simulink model "VGWEC_Model_Final"  (R2022a)
settings: Solver=ode3  StartTime=0.0  StopTime=tSim  FixedStep=dt  RelTol=1e-3
undefined symbols (not defined in the file): amp_Wave, AR3, aRInterp, BR3, bRInterp, CR3, DR3, hydroCoeff, hydroVCoeff, I55, tfRadAR_ROm, tfRadBR_ROm, tfRadCR_ROm, tfRadDR_ROm, theta0, Time_Variant, tRamp, w_Wave, w_WaveIndx, X, Y, Z
libraries: sm_lib x8, nesl_utility x5, cstblocks x4, simulink x2
settings Model: Creator=tdemonte  LastModifiedBy=tdemonte
settings SimscapeCC: EditingMode=Restricted
settings ExplorerConfigSet: InternalSimMechanicsExplorerSettings="<ExplorerConfiguration><canonicalview>default</canonicalview><AnimationSetting><BasePlaybackSpeed>1.0</BasePlaybackSpeed><PlaybackSpeedFactor>1.0</PlaybackSpeedFactor></AnimationSetting><TilePanel><TileInfo><Tiles Columns=\"1\" Count=\"1\" Rows=\"1\"><Column Weight=\"1\"/><Row Weight=\"1\"/><Tile Height=\"1\" Width=\"1\" X=\"0\" Y=\"0\"/></Tiles></TileInfo><SceneInfo><SceneViewer><BGColor><R>0.800000011920928955</R><G>0.800000011920928955</G><B>0.800000011920928955</B></BGColor><Camera><DoPerspective>off</DoPerspective><Position><X>1.56106141432910372</X><Y>-1.5610514773575217</Y><Z>1.56105459035981609</Z></Position><Center><X>9.99552486290526904e-06</X><Y>-5.85532809332417288e-08</Y><Z>3.17155557533474546e-06</Z></Center><Up><X>-0.408248290463863073</X><Y>0.408248290463863073</Y><Z>0.816496580927726145</Z></Up><ViewLimDist>1</ViewLimDist><YLim>1.9911708307266236</YLim><XLim>3.77091781730319342</XLim></Camera></SceneViewer></SceneInfo></TilePanel><MechEditorPanel><Cameras/><GfxPanelCameraMap/><VideoCreator><PlaybackSpeedRatio>1.0</PlaybackSpeedRatio><FrameRate>30</FrameRate><VideoFormat>Motion JPEG AVI</VideoFormat><FrameSize>auto</FrameSize></VideoCreator></MechEditorPanel></ExplorerConfiguration>"

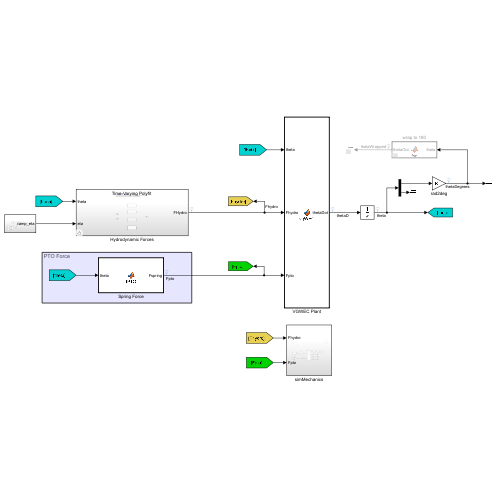
[thumbnail: Simulink's stored preview of the top-level diagram]
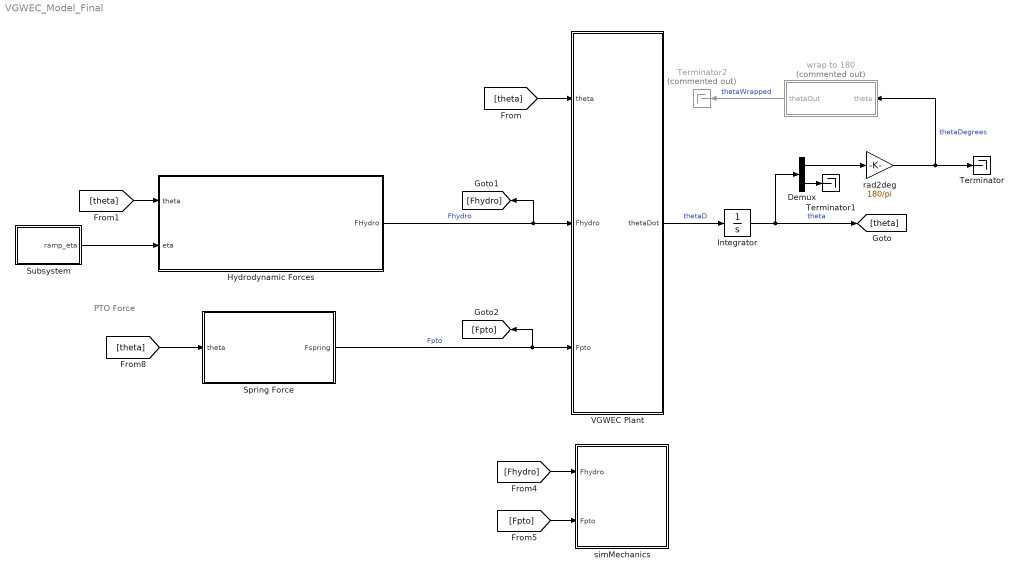
== system VGWEC_Model_Final ==
  note: PTO Force
  Demux : Demux  Outputs=2
  Hydrodynamic Forces : Subsystem  Variant=on
  Integrator : Integrator  InitialCondition=theta0
  Spring Force : MATLAB Function  TreatAsAtomicUnit=on
  Subsystem : Subsystem
  Terminator : Terminator
  Terminator1 : Terminator
  Terminator2 : Terminator  Commented=on
  VGWEC Plant : MATLAB Function  TreatAsAtomicUnit=on
  rad2deg : Gain  Gain=180/pi
  simMechanics : Subsystem
  wrap to 180 : MATLAB Function  Commented=on  TreatAsAtomicUnit=on
  wires:
  VGWEC Plant/1(thetaDot) -> Integrator/1  "thetaD"
  [theta] -> VGWEC Plant/1(theta)
  rad2deg/1 -> Terminator/1, wrap to 180/1(theta)  "thetaDegrees"
  [theta] -> Spring Force/1(theta)
  Spring Force/1(Fspring) -> [Fpto], VGWEC Plant/3(Fpto)  "Fpto"
  [theta] -> Hydrodynamic Forces/1(theta)
  Hydrodynamic Forces/1(FHydro) -> [Fhydro], VGWEC Plant/2(Fhydro)  "Fhydro"
  [Fhydro] -> simMechanics/1(Fhydro)
  [Fpto] -> simMechanics/2(Fpto)
  Integrator/1 -> Demux/1, [theta]  "theta"
  Subsystem/1(ramp_eta) -> Hydrodynamic Forces/2(eta)
  Demux/1 -> rad2deg/1
  Demux/2 -> Terminator1/1
  wrap to 180/1(thetaOut) -> Terminator2/1  "thetaWrapped"

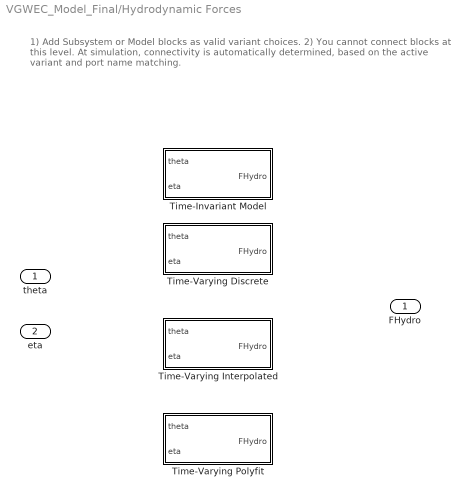
== system VGWEC_Model_Final/Hydrodynamic Forces ==
  note: 1) Add Subsystem or Model blocks as valid variant choices.
      | 2) You cannot connect blocks at this level. At simulation, connectivity is automatically
      | determined, based on the active variant and port name matching.
  theta : Inport
  eta : Inport  Port=2
  Time-Invariant Model : Subsystem  VariantControl=Time_Variant == 0
  "Time-Varying Discrete " : Subsystem  VariantControl=Time_Variant == 1
  Time-Varying Interpolated : Subsystem  VariantControl=Time_Variant == 2
  "Time-Varying Polyfit " : Subsystem  VariantControl=Time_Variant == 3
  FHydro : Outport

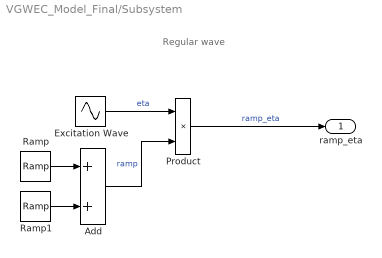
== system VGWEC_Model_Final/Subsystem ==
  note: Regular wave
  Add : Sum
  Excitation Wave : Sin  Amplitude=amp_Wave  Frequency=w_Wave  SampleTime=0
  Product : Product
  Ramp : simulink/Sources/Ramp  slope=1/tRamp  start=0  InitialOutput=0
  Ramp1 : simulink/Sources/Ramp  slope=-1/tRamp  start=tRamp  InitialOutput=0
  ramp_eta : Outport
  wires:
  Add/1 -> Product/2  "ramp"
  Excitation Wave/1 -> Product/1  "eta"
  Ramp1/1 -> Add/2
  Product/1 -> ramp_eta/1  "ramp_eta"
  Ramp/1 -> Add/1

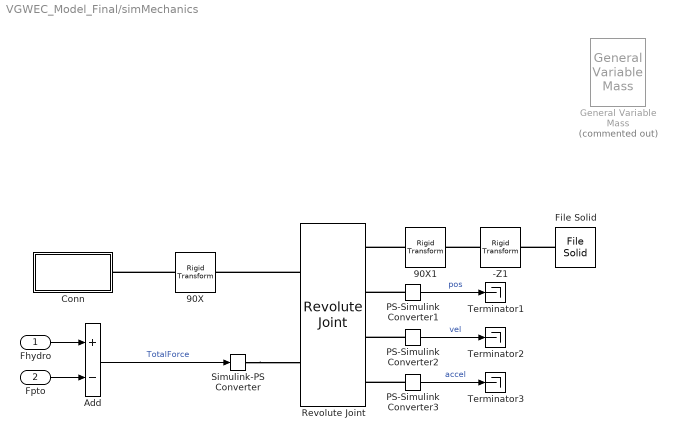
== system VGWEC_Model_Final/simMechanics ==
  Fhydro : Inport
  Fpto : Inport  Port=2
  -Z1 : sm_lib/Frames and Transforms/Rigid Transform  TranslationMethod=StandardAxis  TranslationStandardOffset=1  TranslationLengthUnit=m  TranslationStandardAxis=+Z  TranslationCartesianOffset=[0 0 ]  TranslationROffset=0  TranslationROffsetUnits=m  TranslationZOffset=0  TranslationZOffsetUnits=m  TranslationThetaOffset=0  TranslationThetaOffsetUnits=deg  RotationMethod=None  RotationAngleUnits=deg  RotationStandardAxis=+X  RotationAngle=90  RotationArbitraryAxis=[0 0 1]  FollAlignAxisA=+X  BaseAlignAxisA=+Y  FollAlignAxisB=+Y  BaseAlignAxisB=+Z  RotationSequenceAxes=FollowerAxes  RotationSequence=XYX  RotationSequenceAngles=[0 0 0]  RotationSequenceAnglesUnits=deg  RotationMatrix=[1 0 0; 0 1 0; 0 0 1]
  90X : sm_lib/Frames and Transforms/Rigid Transform  TranslationMethod=None  TranslationStandardOffset=1  TranslationLengthUnit=m  TranslationStandardAxis=-Y  TranslationCartesianOffset=[0 0 ]  TranslationROffset=0  TranslationROffsetUnits=m  TranslationZOffset=0  TranslationZOffsetUnits=m  TranslationThetaOffset=0  TranslationThetaOffsetUnits=deg  RotationMethod=StandardAxis  RotationAngleUnits=deg  RotationStandardAxis=+X  RotationAngle=90  RotationArbitraryAxis=[0 0 1]  FollAlignAxisA=+X  BaseAlignAxisA=+Y  FollAlignAxisB=+Y  BaseAlignAxisB=+Z  RotationSequenceAxes=FollowerAxes  RotationSequence=XYX  RotationSequenceAngles=[0 0 0]  RotationSequenceAnglesUnits=deg  RotationMatrix=[1 0 0; 0 1 0; 0 0 1]
  90X1 : sm_lib/Frames and Transforms/Rigid Transform  TranslationMethod=None  TranslationStandardOffset=0  TranslationLengthUnit=m  TranslationStandardAxis=+Z  TranslationCartesianOffset=[0 -1 0]  TranslationROffset=0  TranslationROffsetUnits=m  TranslationZOffset=0  TranslationZOffsetUnits=m  TranslationThetaOffset=0  TranslationThetaOffsetUnits=deg  RotationMethod=StandardAxis  RotationAngleUnits=deg  RotationStandardAxis=-X  RotationAngle=90  RotationArbitraryAxis=[0 0 1]  FollAlignAxisA=+X  BaseAlignAxisA=+Y  FollAlignAxisB=+Y  BaseAlignAxisB=+Z  RotationSequenceAxes=FollowerAxes  RotationSequence=XYX  RotationSequenceAngles=[0 0 0]  RotationSequenceAnglesUnits=deg  RotationMatrix=[1 0 0; 0 1 0; 0 0 1]
  Add : Sum  Inputs=+-
  Conn : Subsystem
  File Solid : sm_lib/Body Elements/File Solid  ExtGeomFileName=C:\Users\tdemonte\OneDrive - NREL\VGWEC\Full Flap Data\flap0deg.STL  UnitType=Custom  ExtGeomFileUnits=mm  StepReaderType=HEX  ExportConvexHullGeometry=off  InertiaType=Custom  Mass=I55  MassUnits=kg  CenterOfMass=[0 0 -1]  CenterOfMassUnits=m  MomentsOfInertia=[1 hydroVCoeff.IA(hydroCoeff.singleThetaIndex) + hydroCoeff.IQ 1]  MomentsOfInertiaUnits=kg*m^2  ProductsOfInertia=[0 0 0]  ProductsOfInertiaUnits=kg*m^2  BasedOnType=Mass  Density=1000  DensityUnits=kg/m^3  DoExposeReferenceFrame=on  SerializedFrames=<Frames/>  GraphicType=FromGeometry  MarkerShape=Sphere  MarkerSize=10  GraphicVisPropType=SimpleVisualProperties  GraphicDiffuseColor=[0.5 0.5 0.5]  GraphicSpecularColor=[0.5 0.5 0.5 1.0]  GraphicAmbientColor=[0.15 0.15 0.15 1.0]  GraphicEmissiveColor=[0.0 0.0 0.0 1.0]  GraphicShininess=75  GraphicOpacity=0.5
  General Variable Mass : sm_lib/Body Elements/Variable Mass/General Variable Mass  Commented=on  VariableInertiaType=Custom  MassType=TimeVarying  Mass=1  MassUnits=kg  CenterOfMassType=Constant  CenterOfMass=[0 0 0]  CenterOfMassUnits=m  InertiaMatrixType=Constant  MomentsOfInertia=[1 1 1]  MomentsOfInertiaUnits=kg*m^2  ProductsOfInertia=[0 0 0]  ProductsOfInertiaUnits=kg*m^2  GraphicType=InertiaEllipsoid  MarkerShape=Sphere  MarkerSize=10  GraphicVisPropType=SimpleVisualProperties  GraphicDiffuseColor=[0.5 0.5 0.5]  GraphicSpecularColor=[0.5 0.5 0.5 1.0]  GraphicAmbientColor=[0.15 0.15 0.15 1.0]  GraphicEmissiveColor=[0.0 0.0 0.0 1.0]  GraphicShininess=75  GraphicOpacity=1.0
      settings: SourceProductBaseCode=MS
  PS-Simulink Converter1 : nesl_utility/PS-Simulink Converter  PhysicalDomain=network_engine_domain  SubClassName=ps_output  LeftPortType=input  RightPortType=output  PseudoPeriodic=off  Frequencies=[]  VectorFormat=inherit  Unit=inherit  AffineConversion=off
      settings: SourceProductBaseCode=SS,PW,VE
  PS-Simulink Converter2 : nesl_utility/PS-Simulink Converter  PhysicalDomain=network_engine_domain  SubClassName=ps_output  LeftPortType=input  RightPortType=output  PseudoPeriodic=off  Frequencies=[]  VectorFormat=inherit  Unit=inherit  AffineConversion=off
      settings: SourceProductBaseCode=SS,PW,VE
  PS-Simulink Converter3 : nesl_utility/PS-Simulink Converter  PhysicalDomain=network_engine_domain  SubClassName=ps_output  LeftPortType=input  RightPortType=output  PseudoPeriodic=off  Frequencies=[]  VectorFormat=inherit  Unit=inherit  AffineConversion=off
      settings: SourceProductBaseCode=SS,PW,VE
  Revolute Joint : sm_lib/Joints/Revolute Joint  JointMode=Normal  SenseConstraintForce=off  SenseConstraintForceX=off  SenseConstraintForceY=off  SenseConstraintForceZ=off  SenseConstraintTorque=off  SenseConstraintTorqueX=off  SenseConstraintTorqueY=off  SenseConstraintTorqueZ=off  SenseTotalForce=off  SenseTotalForceX=off  SenseTotalForceY=off  SenseTotalForceZ=off  SenseTotalTorque=off  SenseTotalTorqueX=off  SenseTotalTorqueY=off  SenseTotalTorqueZ=off  CompositeWrenchDir=FollowerOnBase  CompositeWrenchFrame=BaseFrame  EquilibriumPosition=0  EquilibriumPositionUnits=deg  SpringStiffness=0  SpringStiffnessUnits=N*m/deg  DampingCoefficient=0  DampingCoefficientUnits=N*m/(deg/s)  TorqueActuationMode=InputTorque  MotionActuationMode=ComputedMotion  SensePosition=on  SenseVelocity=on  SenseAcceleration=on  SenseTorqueForce=off  SenseLowerLimitTorqueForce=off  SenseUpperLimitTorqueForce=off  LowerLimitSpecify=off  LowerLimitBound=-90  LowerLimitBoundUnits=deg  LowerLimitStiffness=1e4  LowerLimitStiffnessUnits=N*m/deg  LowerLimitDamping=10  LowerLimitDampingUnits=N*m/(deg/s)  LowerLimitTransitionRegionWidth=0.1  LowerLimitTransitionRegionWidthUnits=deg  UpperLimitSpecify=off  UpperLimitBound=90  UpperLimitBoundUnits=deg  UpperLimitStiffness=1e4  UpperLimitStiffnessUnits=N*m/deg  UpperLimitDamping=10  UpperLimitDampingUnits=N*m/(deg/s)  UpperLimitTransitionRegionWidth=0.1  UpperLimitTransitionRegionWidthUnits=deg  PositionTargetSpecify=off  PositionTargetPriority=High  PositionTargetValue=0  PositionTargetValueUnits=deg  VelocityTargetSpecify=off  VelocityTargetPriority=High  VelocityTargetValue=0  VelocityTargetValueUnits=deg/s
  Simulink-PS Converter : nesl_utility/Simulink-PS Converter  PhysicalDomain=network_engine_domain  SubClassName=ps_input  LeftPortType=input  RightPortType=output  PseudoPeriodic=off  Frequencies=[]  NoiseDistribution=none  NoiseParameters=[]  Unit=1  AffineConversion=off  FilteringAndDerivatives=provide  SimscapeFilterOrder=1  InputFilterTimeConstant=0.001  UdotUserProvided=0
      settings: SourceProductBaseCode=SS,PW,VE
  Terminator1 : Terminator
  Terminator2 : Terminator
  Terminator3 : Terminator
  wires:
  Add/1 -> Simulink-PS Converter/1  "TotalForce"
  PS-Simulink Converter3/1 -> Terminator3/1  "accel"
  PS-Simulink Converter2/1 -> Terminator2/1  "vel"
  PS-Simulink Converter1/1 -> Terminator1/1  "pos"
  Fhydro/1 -> Add/1
  Fpto/1 -> Add/2
  connections:
  PS-Simulink Converter3/LConn1 -- Revolute Joint/RConn4
  File Solid/RConn1 -- -Z1/RConn1
  PS-Simulink Converter2/LConn1 -- Revolute Joint/RConn3
  PS-Simulink Converter1/LConn1 -- Revolute Joint/RConn2
  Simulink-PS Converter/RConn1 -- Revolute Joint/LConn2
  Revolute Joint/LConn1 -- 90X/RConn1
  90X1/LConn1 -- Revolute Joint/RConn1
  90X/LConn1 -- Conn/RConn1
  -Z1/LConn1 -- 90X1/RConn1

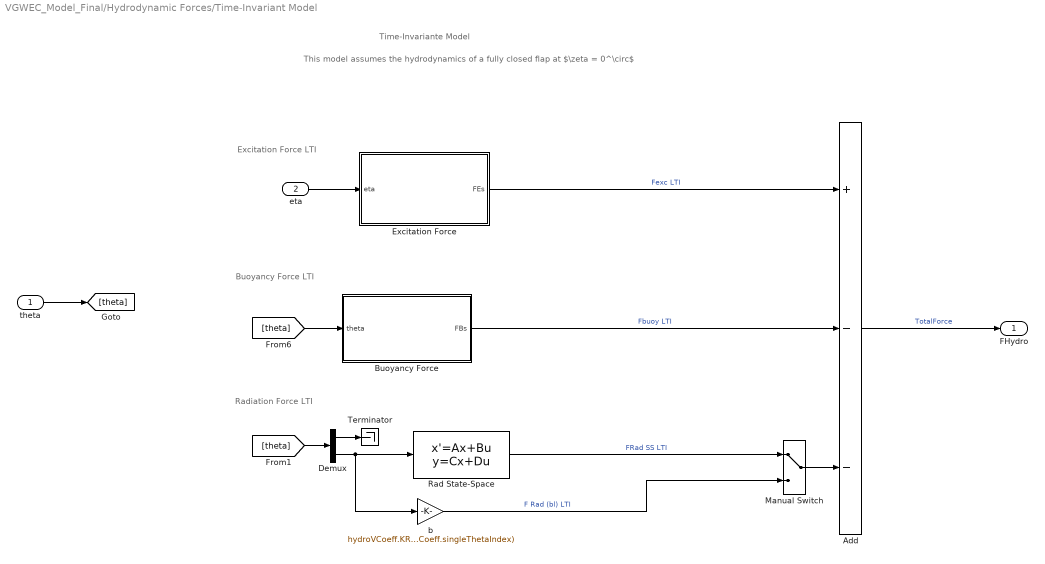
== system VGWEC_Model_Final/Hydrodynamic Forces/Time-Invariant Model ==
  note: Time-Invariante Model
  note: Excitation Force LTI
  note: Radiation Force LTI
  note: Buoyancy Force LTI
  note: This model assumes the hydrodynamics of a fully closed flap at $\zeta = 0^\circ$
  theta : Inport
  eta : Inport  Port=2
  Add : Sum  Inputs=+--
  Buoyancy Force : MATLAB Function  TreatAsAtomicUnit=on
  Demux : Demux  Outputs=2
  "Excitation Force " : MATLAB Function  TreatAsAtomicUnit=on
  Manual Switch : ManualSwitch
  Rad State-Space : StateSpace  A=AR3  B=BR3  C=CR3  D=DR3  InitialCondition=0
  Terminator : Terminator
  b : Gain  Gain=hydroVCoeff.KR(w_WaveIndx, hydroCoeff.singleThetaIndex)
  FHydro : Outport
  wires:
  "Excitation Force "/1(FEs) -> Add/1  "Fexc LTI"
  Demux/2 -> b/1, Rad State-Space/1
  Buoyancy Force/1(FBs) -> Add/2  "Fbuoy LTI"
  eta/1 -> "Excitation Force "/1(eta)
  theta/1 -> [theta]
  [theta] -> Buoyancy Force/1(theta)
  Rad State-Space/1 -> Manual Switch/1  "FRad SS LTI"
  Demux/1 -> Terminator/1
  [theta] -> Demux/1
  Add/1 -> FHydro/1  "TotalForce"
  b/1 -> Manual Switch/2  "F Rad (bl) LTI"
  Manual Switch/1 -> Add/3

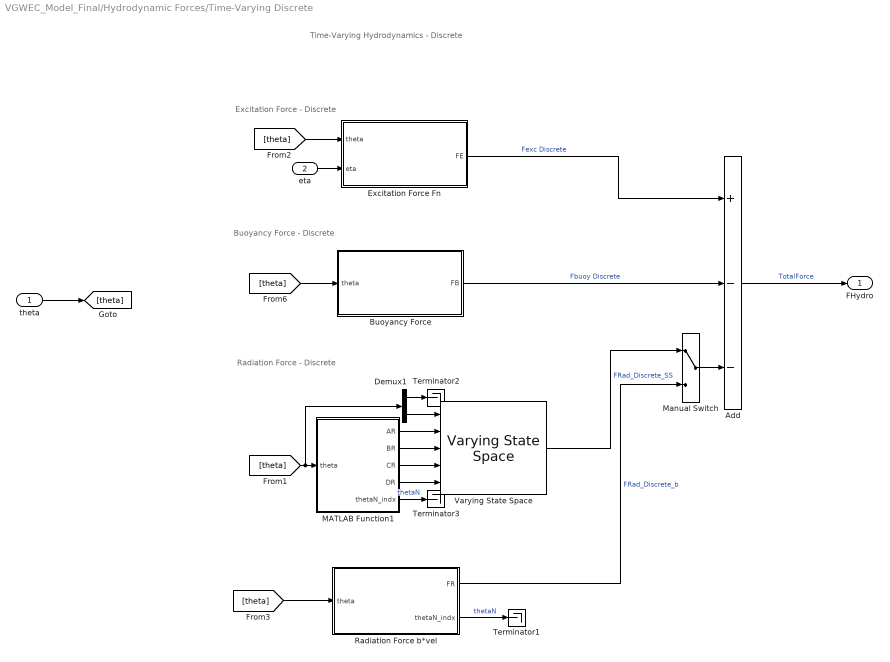
== system VGWEC_Model_Final/Hydrodynamic Forces/Time-Varying Discrete  ==
  note: Buoyancy Force - Discrete
  note: Excitation Force - Discrete
  note: Time-Varying Hydrodynamics - Discrete
  note: Radiation Force - Discrete
  theta : Inport
  eta : Inport  Port=2
  Add : Sum  Inputs=+--
  Buoyancy Force : MATLAB Function  TreatAsAtomicUnit=on
  Demux1 : Demux  Outputs=2
  Excitation Force Fn : MATLAB Function  TreatAsAtomicUnit=on
  MATLAB Function1 : MATLAB Function  TreatAsAtomicUnit=on
  Manual Switch : ManualSwitch
  Radiation Force b*vel : MATLAB Function  TreatAsAtomicUnit=on
  Terminator1 : Terminator
  Terminator2 : Terminator
  Terminator3 : Terminator
  Varying State Space : cstblocks/Linear Parameter Varying/Varying State Space  x0=0  xNames=''  OutputX=off  OutputDX=off
  FHydro : Outport
  wires:
  eta/1 -> Excitation Force Fn/2(eta)
  Buoyancy Force/1(FB) -> Add/2  "Fbuoy Discrete"
  Excitation Force Fn/1(FE) -> Add/1  "Fexc Discrete"
  Add/1 -> FHydro/1  "TotalForce"
  theta/1 -> [theta]
  [theta] -> Excitation Force Fn/1(theta)
  [theta] -> Buoyancy Force/1(theta)
  Demux1/2 -> Varying State Space/1
  Varying State Space/1 -> Manual Switch/1  "FRad_Discrete_SS"
  [theta] -> Demux1/1, MATLAB Function1/1(theta)
  [theta] -> Radiation Force b*vel/1(theta)
  MATLAB Function1/5(thetaN_indx) -> Terminator3/1  "thetaN"
  MATLAB Function1/2(BR) -> Varying State Space/3
  MATLAB Function1/1(AR) -> Varying State Space/2
  MATLAB Function1/3(CR) -> Varying State Space/4
  Radiation Force b*vel/1(FR) -> Manual Switch/2  "FRad_Discrete_b"
  Demux1/1 -> Terminator2/1
  MATLAB Function1/4(DR) -> Varying State Space/5
  Manual Switch/1 -> Add/3
  Radiation Force b*vel/2(thetaN_indx) -> Terminator1/1  "thetaN"

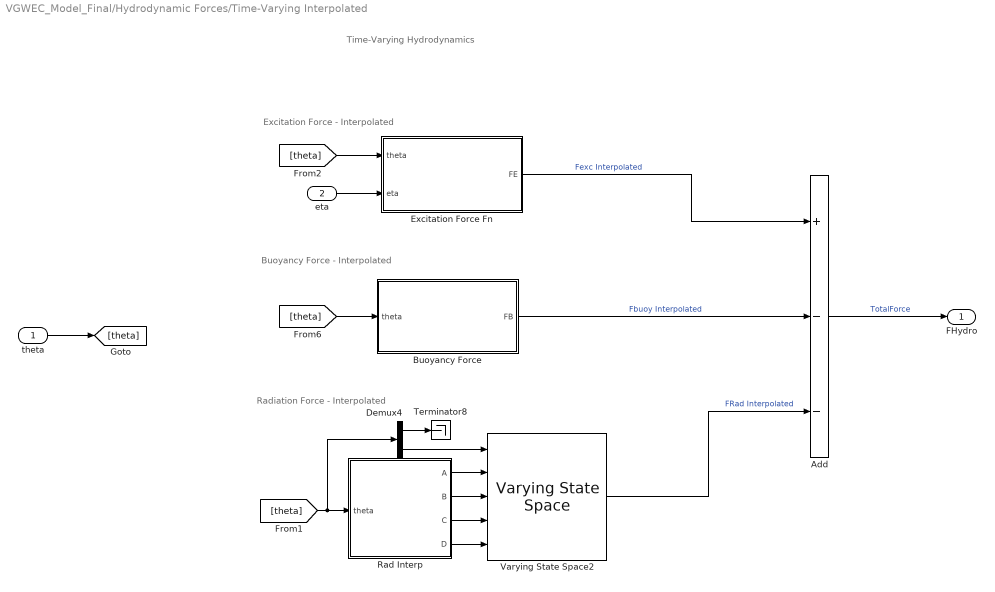
== system VGWEC_Model_Final/Hydrodynamic Forces/Time-Varying Interpolated ==
  note: Radiation Force - Interpolated
  note: Time-Varying Hydrodynamics
  note: Excitation Force - Interpolated
  note: Buoyancy Force - Interpolated
  theta : Inport
  eta : Inport  Port=2
  Add : Sum  Inputs=+--
  Buoyancy Force : MATLAB Function  TreatAsAtomicUnit=on
  Demux4 : Demux  Outputs=2
  Excitation Force Fn : MATLAB Function  TreatAsAtomicUnit=on
  Rad Interp : MATLAB Function  TreatAsAtomicUnit=on
  Terminator8 : Terminator
  Varying State Space2 : cstblocks/Linear Parameter Varying/Varying State Space  x0=0  xNames=''  OutputX=off  OutputDX=off
  FHydro : Outport
  wires:
  [theta] -> Buoyancy Force/1(theta)
  [theta] -> Excitation Force Fn/1(theta)
  theta/1 -> [theta]
  Add/1 -> FHydro/1  "TotalForce"
  Excitation Force Fn/1(FE) -> Add/1  "Fexc Interpolated"
  Buoyancy Force/1(FB) -> Add/2  "Fbuoy Interpolated"
  eta/1 -> Excitation Force Fn/2(eta)
  Demux4/2 -> Varying State Space2/1
  Rad Interp/3(C) -> Varying State Space2/4
  Rad Interp/1(A) -> Varying State Space2/2
  Demux4/1 -> Terminator8/1
  Rad Interp/2(B) -> Varying State Space2/3
  Rad Interp/4(D) -> Varying State Space2/5
  [theta] -> Demux4/1, Rad Interp/1(theta)
  Varying State Space2/1 -> Add/3  "FRad Interpolated"

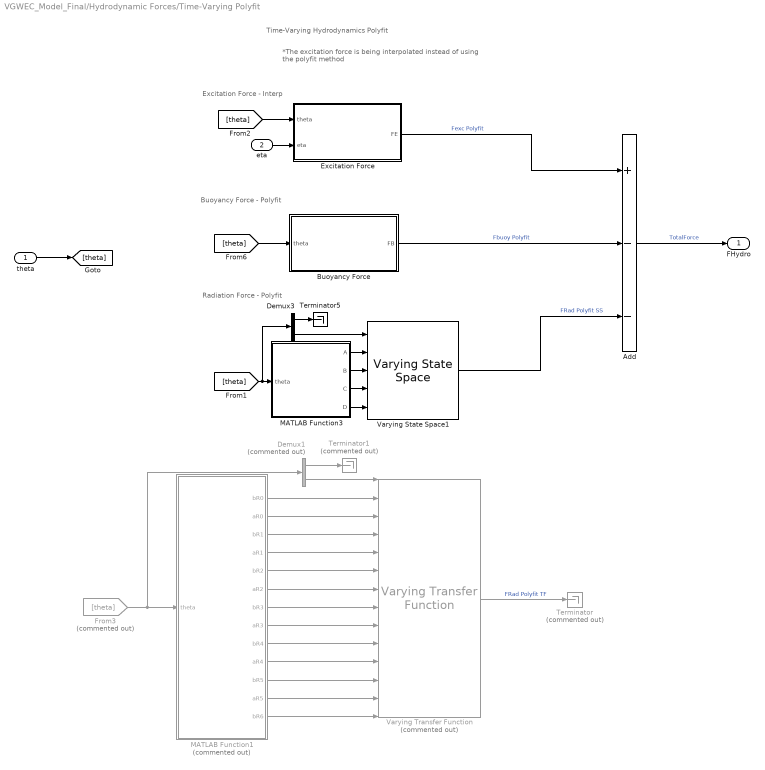
== system VGWEC_Model_Final/Hydrodynamic Forces/Time-Varying Polyfit  ==
  note: Radiation Force - Polyfit
  note: Time-Varying Hydrodynamics Polyfit
  note: Excitation Force - Interp
  note: Buoyancy Force - Polyfit
  note: *The excitation force is being interpolated instead of using the polyfit method
  theta : Inport
  eta : Inport  Port=2
  Add : Sum  Inputs=+--
  Buoyancy Force : MATLAB Function  TreatAsAtomicUnit=on
  Demux1 : Demux  Commented=on  Outputs=2
  Demux3 : Demux  Outputs=2
  Excitation Force : MATLAB Function  TreatAsAtomicUnit=on
  From3 : From  Commented=on  GotoTag=theta
  MATLAB Function1 : MATLAB Function  Commented=on  TreatAsAtomicUnit=on
  MATLAB Function3 : MATLAB Function  TreatAsAtomicUnit=on
  Terminator : Terminator  Commented=on
  Terminator1 : Terminator  Commented=on
  Terminator5 : Terminator
  Varying State Space1 : cstblocks/Linear Parameter Varying/Varying State Space  x0=0  xNames=''  OutputX=off  OutputDX=off
  Varying Transfer Function : cstblocks/Linear Parameter Varying/Varying Transfer Function  Commented=on  N=6
  FHydro : Outport
  wires:
  [theta] -> Buoyancy Force/1(theta)
  [theta] -> Excitation Force/1(theta)
  theta/1 -> [theta]
  Add/1 -> FHydro/1  "TotalForce"
  Excitation Force/1(FE) -> Add/1  "Fexc Polyfit"
  Buoyancy Force/1(FB) -> Add/2  "Fbuoy Polyfit"
  eta/1 -> Excitation Force/2(eta)
  Demux3/2 -> Varying State Space1/1
  Varying State Space1/1 -> Add/3  "FRad Polyfit SS"
  MATLAB Function3/4(D) -> Varying State Space1/5
  MATLAB Function3/1(A) -> Varying State Space1/2
  Demux3/1 -> Terminator5/1
  MATLAB Function3/2(B) -> Varying State Space1/3
  MATLAB Function3/3(C) -> Varying State Space1/4
  [theta] -> Demux3/1, MATLAB Function3/1(theta)
  MATLAB Function1/1(bR0) -> Varying Transfer Function/2
  MATLAB Function1/2(aR0) -> Varying Transfer Function/3
  MATLAB Function1/3(bR1) -> Varying Transfer Function/4
  MATLAB Function1/4(aR1) -> Varying Transfer Function/5
  MATLAB Function1/5(bR2) -> Varying Transfer Function/6
  MATLAB Function1/6(aR2) -> Varying Transfer Function/7
  MATLAB Function1/7(bR3) -> Varying Transfer Function/8
  MATLAB Function1/8(aR3) -> Varying Transfer Function/9
  MATLAB Function1/9(bR4) -> Varying Transfer Function/10
  MATLAB Function1/10(aR4) -> Varying Transfer Function/11
  MATLAB Function1/11(bR5) -> Varying Transfer Function/12
  MATLAB Function1/12(aR5) -> Varying Transfer Function/13
  MATLAB Function1/13(bR6) -> Varying Transfer Function/14
  Demux1/2 -> Varying Transfer Function/1
  From3/1 -> Demux1/1, MATLAB Function1/1(theta)
  Demux1/1 -> Terminator1/1
  Varying Transfer Function/1 -> Terminator/1  "FRad Polyfit TF"

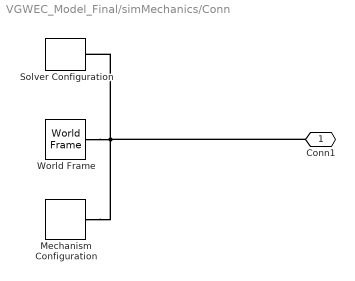
== system VGWEC_Model_Final/simMechanics/Conn ==
  Mechanism Configuration : sm_lib/Utilities/Mechanism Configuration  UniformGravity=Constant  GravityVector=[0 0 -9.80665]  GravityUnits=m/s^2  LinearizationDelta=0.001  JointModeTransitionNonlinearIterations=2
  Solver Configuration : nesl_utility/Solver Configuration  PhysicalDomain=network_engine_domain  SubClassName=solver  LeftPortType=input  RightPortType=generic  Tones=[]  Harmonics=[]  SimulateNoise=off  Profile=off  UseLocalSampling=off  EnableSwitchedLinearOptims=on  FrequencyDomain=off  UseCCode=off  RelTol=0.001  AbsTol=1e-06  MinStep=1e-09  ToWorkspace=off  RevertToSquareIcSolve=off  NumHomotopyIterations=100  PhasorMode=off  PhasorModeNumHarmonics=1  IndexReductionMethod=DerivativeReplacement  DoDC=off  ResidualTolerance=1e-09  UseLocalSolver=off  LocalSolverChoice=NE_BACKWARD_EULER_ADVANCER  LocalSolverSampleTime=0.001  DoFixedCost=off  MaxNonlinIter=3  MaxModeIter=2  ComputeImpulses=off  ImpulseIterations=2  LinearAlgebra=Sparse  LinearAlgebraNumThread=0  EquationFormulation=NE_TIME_EF  DelaysMemoryBudget=1024  AutomaticFiltering=on  FilteringTimeConstant=0.001  PartitionStorageMethod=AS_NEEDED  PartitionMemoryBudget=1024  PartitionMethod=FAST
      settings: SourceProductBaseCode=SS,PW,VE
  World Frame : sm_lib/Frames and Transforms/World Frame
  Conn1 : PMIOPort  Side=Right
  connections:
  World Frame/RConn1 -- Solver Configuration/RConn1 -- Mechanism Configuration/RConn1 -- Conn1/RConn1

== matlab function VGWEC_Model_Final/Hydrodynamic Forces/Time-Varying Polyfit /MATLAB Function3 ==
  data: theta input; A output size=[6 6]; B output size=[6 1]; hydroVCoeff parameter; C output size=[1 6]; D output size=1
function [A,B,C,D] = RadTFCoeffs(theta, hydroVCoeff)
% This function extracts the coefficients of the Radiation Transfer
% Function based on previously fitted data between discretized thetas. 

% Inputs: 
% theta0      = current states condition
% hydrovCoeff = time-variable hydrodynamic coefficients
% thetaN      = pitch angle index

% Outputs: 
% bR    = numerator 
% aR    = denominator 

% States: 
theta1  = theta(1); % (1) theta:  pitch angle response
% theta2  = theta(2); % (2) thetaD: pitch angle velocity

theta1 = wrapToPi(theta1); 
theta1D = rad2deg(theta1); 
% Find the index for the discretized theta 
if abs(theta1D) >= 95
    theta1D = 180 - abs(theta1D);
end 

% % Get transfer function coefficients depending on the discretized angle. 
aR       = zeros(1,7); 
bR       = zeros(1,7);

theta1D = abs(theta1D); 

aR(1)    = 1; % But no lead denominator
aR(2)    = polyval(hydroVCoeff.aRFit(2,:), theta1D,[], hydroVCoeff.aR_mu(2,:));
aR(3)    = polyval(hydroVCoeff.aRFit(3,:), theta1D,[], hydroVCoeff.aR_mu(3,:));
aR(4)    = polyval(hydroVCoeff.aRFit(4,:), theta1D,[], hydroVCoeff.aR_mu(4,:));
aR(5)    = polyval(hydroVCoeff.aRFit(5,:), theta1D,[], hydroVCoeff.aR_mu(5,:));
aR(6)    = polyval(hydroVCoeff.aRFit(6,:), theta1D,[], hydroVCoeff.aR_mu(6,:));
aR(7)    = polyval(hydroVCoeff.aRFit(7,:), theta1D,[], hydroVCoeff.aR_mu(7,:));

bR(1)    = polyval(hydroVCoeff.bRFit(1,:), theta1D,[], hydroVCoeff.bR_mu(1,:));
bR(2)    = polyval(hydroVCoeff.bRFit(2,:), theta1D,[], hydroVCoeff.bR_mu(2,:));
bR(3)    = polyval(hydroVCoeff.bRFit(3,:), theta1D,[], hydroVCoeff.bR_mu(3,:));
bR(4)    = polyval(hydroVCoeff.bRFit(4,:), theta1D,[], hydroVCoeff.bR_mu(4,:));
bR(5)    = polyval(hydroVCoeff.bRFit(5,:), theta1D,[], hydroVCoeff.bR_mu(5,:));
bR(6)    = polyval(hydroVCoeff.bRFit(6,:), theta1D,[], hydroVCoeff.bR_mu(6,:));
bR(7)    = polyval(hydroVCoeff.bRFit(7,:), theta1D,[], hydroVCoeff.bR_mu(7,:));

% % Get transfer function coefficients depending on the discretized angle. 
A       = zeros(6,6); 
B       = zeros(6,1); 
C       = zeros(1,6); 
D       = 0; 

[A(:,:), B(:,1), C(1,:), D(1)] = tf2ss(bR,aR);

== matlab function VGWEC_Model_Final/Hydrodynamic Forces/Time-Varying Polyfit /Buoyancy Force ==
  data: theta input size=[1 2]; FB output double size=1; hydroVCoeff parameter
function FB = fBuoy(theta, hydroVCoeff)

% States: 
theta1  = theta(1); % (1) theta:  pitch angle response
% theta2  = theta(2); % (2) thetaD: pitch angle velocity

theta1 = wrapToPi(theta1); 
theta1D = rad2deg(theta1); 
% Find the index for the discretized theta 
if abs(theta1D) >= 95
    theta1D = 180 - abs(theta1D);
end 

c  = zeros(1,1); 
c  = polyval(hydroVCoeff.cFit, abs(theta1D),[], hydroVCoeff.c_mu); % Hydrostatic restoring coefficient. (t) 

FB    = 0; 
FB(1) = c*theta1; % Buoyancy Force for Time-Varying Hydrodynamics (N)

== matlab function VGWEC_Model_Final/Hydrodynamic Forces/Time-Varying Polyfit /Excitation Force ==
  data: theta input size=[1 2]; FE output double size=1; eta input size=1; hydroCoeff parameter; hydroVCoeff parameter; w_Wave parameter
function FE= fE(theta,eta,hydroCoeff, hydroVCoeff, w_Wave)
% This function generates the linear excitation force

% Inputs: 
% theta       = current states condition
% eta         = wave excitation (m)
% w_Wave      = wave excitation angular frequency 'Omega' (rad/s)
% hydroCoeff  = time-invariable hydrodynamic coefficients
% hydrovCoeff = time-variable hydrodynamic coefficients


% Outputs: 
% FE    = excitation force (N) 
theta1 = theta(1); 

% Find the index for the discretized theta 
theta1N = wrapToPi(theta1); 

if abs(rad2deg(theta1N)) >= 95 
    theta1N = pi - abs(theta1N); 
end 

thetaN = find(deg2rad(hydroCoeff.fineTheta) > abs(theta1N),1); 


% Find the index for the wave excitation frequency 
w  = find(hydroCoeff.w > w_Wave,1)-1;


KE = hydroVCoeff.FExcInterp(w, thetaN); % Added mass moment of inertia at inf. freq. (t)

FE = zeros(1,1); 
FE(1) = eta*KE;

== matlab function VGWEC_Model_Final/Hydrodynamic Forces/Time-Varying Discrete /Buoyancy Force ==
  data: theta input size=[1 2]; FB output double size=1; hydroCoeff parameter; hydroVCoeff parameter
function FB = fBuoy(theta,hydroCoeff, hydroVCoeff)
% % This is the buoyancy force function

% States: 
theta1  = theta(1); % (1) theta:  pitch angle response
% theta2  = theta(2); % (2) thetaD: pitch angle velocity

% Find the index for the discretized theta 

theta1N = wrapToPi(theta1); 

if abs(rad2deg(theta1N)) >= 95 
    theta1N = pi - abs(theta1N);
end 


thetaN = find(deg2rad(hydroCoeff.theta) > abs(theta1N),1); 

c  = hydroVCoeff.c(thetaN); % Hydrostatic restoring coefficient. (t) 
FB = 0; 
FB(1) = c*theta1; % Buoyancy Force for Time-Varying Hydrodynamics (N)

== matlab function VGWEC_Model_Final/Hydrodynamic Forces/Time-Invariant Model/Buoyancy Force ==
  data: theta input size=[1 2]; FBs output double size=1; hydroCoeff parameter; hydroVCoeff parameter
function FBs = fBuoy(theta,hydroCoeff, hydroVCoeff)

% States: 
theta1  = theta(1); % (1) theta:  pitch angle response
% theta2  = theta(2); % (2) thetaD: pitch angle velocity

% Find the index for the discretized theta 
% if abs(rad2deg(theta1)) > 100
%     theta1 = 180 - abs(rad2deg(theta1));
%     theta1 = deg2rad(theta1);
% end 

%% Constant Theta
cs  = hydroVCoeff.c(hydroCoeff.singleThetaIndex); % Hydrostatic restoring coefficient. (t) 
FBs = 0; 
FBs(1) = cs*theta1;

== matlab function VGWEC_Model_Final/Hydrodynamic Forces/Time-Varying Discrete /Excitation Force Fn ==
  data: theta input size=[1 2]; FE output double size=1; eta input size=1; hydroCoeff parameter; hydroVCoeff parameter; w_Wave parameter
function FE= fE(theta,eta,hydroCoeff, hydroVCoeff, w_Wave)

% % Declare the excitation force function as an extrinsic function
% %coder.extrinsic('fExc');
% 
% FE = fExc(theta, eta, w_Wave,hydroVCoeff,hydroCoeff);
% 
% function FE = fExc(theta, eta, w_Wave,hydroVCoeff,hydroCoeff)
% This function generates the linear excitation force

% Inputs: 
% theta0      = current states condition
% eta         = wave excitation (m)
% w_Wave      = wave excitation angular frequency 'Omega' (rad/s)
% hydroCoeff  = time-invariable hydrodynamic coefficients
% hydrovCoeff = time-variable hydrodynamic coefficients


% Outputs: 
% FE    = excitation force (N) 
theta1 = theta(1); 

theta1N = wrapToPi(theta1); 

if abs(rad2deg(theta1N)) >= 95 
    theta1N = pi - abs(theta1N); 
end 

theta1Ndeg = rad2deg(theta1N);

thetaN = find(deg2rad(hydroCoeff.theta) > abs(theta1N),1); 


% Find the index for the wave excitation frequency 
w  = find(hydroCoeff.w > w_Wave,1)-1;

KE = hydroVCoeff.KE(w, thetaN); % Added mass moment of inertia at inf. freq. (t)

FE = zeros(1,1); 
FE(1) = eta*KE;

== matlab function VGWEC_Model_Final/Hydrodynamic Forces/Time-Varying Discrete /MATLAB Function1 ==
  data: theta input; AR output size=[6 6]; BR output size=[6 1]; CR output size=[1 6]; DR output size=1; hydroCoeff parameter; tfRadAR_ROm parameter; tfRadBR_ROm parameter; tfRadCR_ROm parameter; tfRadDR_ROm parameter; thetaN_indx output size=1
function [AR, BR, CR, DR, thetaN_indx] = RadTFCoeffs(theta,hydroCoeff, tfRadAR_ROm, tfRadBR_ROm, tfRadCR_ROm, tfRadDR_ROm)
% This function extracts the coefficients of the Radiation Transfer
% Function based on discrete thetas. 

% Inputs: 
% theta0      = current states condition
% hydrovCoeff = time-variable hydrodynamic coefficients
% thetaN      = pitch angle index

% Outputs: 
% bR    = radiation force (N) 

theta1 = theta(1); 
% Find the index for the discretized theta 
theta1N = wrapToPi(theta1); 

if abs(rad2deg(theta1N)) >= 95 
    theta1N = pi - abs(theta1N);
end 

 
thetaN = find(deg2rad(hydroCoeff.theta) > abs(theta1N),1); 

% % Get transfer function coefficients depending on the discretized angle. 
AR       = zeros(6,6); 
BR       = zeros(6,1); 
CR       = zeros(1,6); 
DR       = 0; 

thetaN_indx = 0; 
thetaN_indx = thetaN(1);

AR(:,:)       = tfRadAR_ROm(:,(thetaN_indx-1)*6+1:(thetaN_indx*6)); % A Matrix Coefficients

BR(:,1)       = tfRadBR_ROm(:,thetaN_indx); % A Matrix Coefficients
CR(1,:)       = tfRadCR_ROm(1,(thetaN_indx-1)*6+1:(thetaN_indx*6)); % A Matrix Coefficients
DR(1)         = tfRadDR_ROm(thetaN_indx); % A Matrix Coefficients

== matlab function VGWEC_Model_Final/Spring Force ==
  data: theta input size=2; Fspring output size=1; hydroCoeff parameter
function Fspring = fPTO(theta,hydroCoeff)

% This function represents the plant of a variable geometry wave energy
% converter. The model here is derived by Mcabe 2006. 

% Inputs: 
% theta      = initial state conditions
% hydroCoeff  = time-invariable hydrodynamic coefficients

% Outputs: 
% Fspring   = PTO spring force

% States: 
theta1  = theta(1); % (1) theta:  pitch angle response
% theta2  = theta(2); % (2) thetaD: pitch angle velocity

% Spring Force to keep the flap from rotating
K       = hydroCoeff.Kspring;  % Spring Constant
Fspring = K * theta1; 

end

== matlab function VGWEC_Model_Final/Hydrodynamic Forces/Time-Varying Discrete /Radiation Force b*vel ==
  data: theta input size=[1 2]; FR output double size=1; hydroCoeff parameter; hydroVCoeff parameter; w_WaveIndx parameter; thetaN_indx output
function [FR, thetaN_indx] = fRad(theta,hydroCoeff, hydroVCoeff,w_WaveIndx)

% States: 
theta1  = theta(1); % (1) theta:  pitch angle response
theta2  = theta(2); % (2) thetaD: pitch angle velocity

% Find the index for the discretized theta 

theta1N = wrapToPi(theta1); 

if abs(rad2deg(theta1N)) >= 95 
    theta1N = pi - abs(theta1N);
end 


thetaN = find(deg2rad(hydroCoeff.theta) > abs(theta1N),1); 

thetaN_indx = 0; 
thetaN_indx = thetaN(1);

b  = hydroVCoeff.KR(w_WaveIndx,thetaN); % Radiation Damping Coefficient  

FR = 0; 
FR(1) = b*theta2; % Buoyancy Force for Time-Varying Hydrodynamics (N)

== matlab function VGWEC_Model_Final/Hydrodynamic Forces/Time-Invariant Model/Excitation Force  ==
  data: eta input size=1; hydroCoeff parameter; hydroVCoeff parameter; w_Wave parameter; FEs output size=1
function  FEs = fE(eta,hydroCoeff, hydroVCoeff, w_Wave)


%% Calculate the Excitation Force for a Constant theta
w  = find(hydroCoeff.w > w_Wave,1)-1;
KE = hydroVCoeff.KE(w, hydroCoeff.singleThetaIndex); % Excitation Force Kernel

FEs = 0; 
FEs(1) = eta*KE;

== matlab function VGWEC_Model_Final/wrap to 180 ==
  data: theta input; thetaOut output
function thetaOut = fcn(theta)

thetaOut = 0; 
thetaOut(1) = wrapTo180(theta);

thetaOut = theta;

== matlab function VGWEC_Model_Final/VGWEC Plant ==
  data: theta input size=2; thetaDot output size=[1 2]; Fhydro input size=1; hydroVCoeff parameter; hydroCoeff parameter; Fpto input; Time_Variant parameter
function thetaDot = vgWEC(theta, Fhydro, hydroVCoeff, hydroCoeff, Fpto, Time_Variant)

% Declare the plant as an extrinsic function
%coder.extrinsic('vgWecPlant_Final');

thetaDot = vgWecPlant_Final(theta, hydroCoeff, hydroVCoeff, Fhydro, Fpto, Time_Variant);

== matlab function VGWEC_Model_Final/Hydrodynamic Forces/Time-Varying Polyfit /MATLAB Function1 ==
  data: theta input; bR0 output size=1; aR0 output size=1; bR1 output size=1; aR1 output size=1; hydroVCoeff parameter; bR2 output size=1; aR2 output size=1; bR3 output size=1; aR3 output size=1; bR4 output size=1; aR4 output size=1; bR5 output size=1; aR5 output size=1; bR6 output size=1
function [bR0,aR0, bR1,aR1, bR2,aR2, bR3,aR3, bR4,aR4, bR5,aR5, bR6]    = RadTFCoeffs(theta, hydroVCoeff)
% This function extracts the coefficients of the Radiation Transfer
% Function based on previously fitted data between discretized thetas. 

% Inputs: 
% theta0      = current states condition
% hydrovCoeff = time-variable hydrodynamic coefficients
% thetaN      = pitch angle index

% Outputs: 
% bR    = numerator 
% aR    = denominator 

% States: 
theta1  = theta(1); % (1) theta:  pitch angle response
% theta2  = theta(2); % (2) thetaD: pitch angle velocity

theta1  = wrapToPi(theta1); 
theta1D = rad2deg(theta1); 
% Find the index for the discretized theta 
if abs(theta1D) >= 95
    theta1D = 180 - abs(theta1D);
end 

% % Get transfer function coefficients depending on the discretized angle. 
theta1D = abs(theta1D); 

% Initialize Data 
aR1    = 0;
aR2    = 0;
aR3    = 0;
aR4    = 0;
aR5    = 0;


bR0    = 0;
bR1    = 0;
bR2    = 0;
bR3    = 0;
bR4    = 0;
bR5    = 0;
bR6    = 0;


% aR0    = 1; % But no lead denominator
aR0    = polyval(hydroVCoeff.aRFit(2,:), theta1D,[], hydroVCoeff.aR_mu(2,:));
aR1    = polyval(hydroVCoeff.aRFit(3,:), theta1D,[], hydroVCoeff.aR_mu(3,:));
aR2    = polyval(hydroVCoeff.aRFit(4,:), theta1D,[], hydroVCoeff.aR_mu(4,:));
aR3    = polyval(hydroVCoeff.aRFit(5,:), theta1D,[], hydroVCoeff.aR_mu(5,:));
aR4    = polyval(hydroVCoeff.aRFit(6,:), theta1D,[], hydroVCoeff.aR_mu(6,:));
aR5    = polyval(hydroVCoeff.aRFit(7,:), theta1D,[], hydroVCoeff.aR_mu(7,:));

bR0    = polyval(hydroVCoeff.bRFit(1,:), theta1D,[], hydroVCoeff.bR_mu(1,:));
bR1    = polyval(hydroVCoeff.bRFit(2,:), theta1D,[], hydroVCoeff.bR_mu(2,:));
bR2    = polyval(hydroVCoeff.bRFit(3,:), theta1D,[], hydroVCoeff.bR_mu(3,:));
bR3    = polyval(hydroVCoeff.bRFit(4,:), theta1D,[], hydroVCoeff.bR_mu(4,:));
bR4    = polyval(hydroVCoeff.bRFit(5,:), theta1D,[], hydroVCoeff.bR_mu(5,:));
bR5    = polyval(hydroVCoeff.bRFit(6,:), theta1D,[], hydroVCoeff.bR_mu(6,:));
bR6    = polyval(hydroVCoeff.bRFit(7,:), theta1D,[], hydroVCoeff.bR_mu(7,:));

== matlab function VGWEC_Model_Final/Hydrodynamic Forces/Time-Varying Interpolated/Buoyancy Force ==
  data: theta input size=[1 2]; FB output double size=1; hydroCoeff parameter; hydroVCoeff parameter
function FB = fBuoy(theta,hydroCoeff, hydroVCoeff)

% States: 
theta1  = theta(1); % (1) theta:  pitch angle response
% theta2  = theta(2); % (2) thetaD: pitch angle velocity

% Find the index for the discretized theta 
theta1N = wrapToPi(theta1); 

if abs(rad2deg(theta1N)) >= 95 
    theta1N = pi - abs(theta1N);
end 

thetaN = find(deg2rad(hydroCoeff.fineTheta) > abs(theta1N),1); 


%% Interpolation
c  = hydroVCoeff.cInterp(thetaN); % Hydrostatic restoring coefficient. (t) 
FB = 0; 
FB(1) = c*theta1; % Buoyancy Force for Time-Varying Hydrodynamics (N)

== matlab function VGWEC_Model_Final/Hydrodynamic Forces/Time-Varying Interpolated/Excitation Force Fn ==
  data: theta input size=[1 2]; FE output double size=1; eta input size=1; hydroCoeff parameter; hydroVCoeff parameter; w_Wave parameter
function FE= fE(theta,eta,hydroCoeff, hydroVCoeff, w_Wave)
% This function generates the linear excitation force

% Inputs: 
% theta       = current states condition
% eta         = wave excitation (m)
% w_Wave      = wave excitation angular frequency 'Omega' (rad/s)
% hydroCoeff  = time-invariable hydrodynamic coefficients
% hydrovCoeff = time-variable hydrodynamic coefficients


% Outputs: 
% FE    = excitation force (N) 
theta1 = theta(1); 

% Find the index for the discretized theta 
theta1N = wrapToPi(theta1); 

if abs(rad2deg(theta1N)) >= 95 
    theta1N = pi - abs(theta1N); 
end 

thetaN = find(deg2rad(hydroCoeff.fineTheta) > abs(theta1N),1); 


% Find the index for the wave excitation frequency 
w  = find(hydroCoeff.w > w_Wave,1)-1;


KE = hydroVCoeff.FExcInterp(w, thetaN); % Added mass moment of inertia at inf. freq. (t)

FE = zeros(1,1); 
FE(1) = eta*KE;

== matlab function VGWEC_Model_Final/Hydrodynamic Forces/Time-Varying Interpolated/Rad Interp ==
  data: theta input; A output size=[6 6]; B output size=[6 1]; hydroCoeff parameter; C output size=[1 6]; D output size=1; aRInterp parameter; bRInterp parameter
function [A,B,C,D] = RadTFCoeffs(theta, hydroCoeff, aRInterp, bRInterp)
% This function extracts the coefficients of the Radiation Transfer
% Function based on previously fitted data between discretized thetas. 

% Inputs: 
% theta0      = current states condition
% hydrovCoeff = time-variable hydrodynamic coefficients
% thetaN      = pitch angle index

% Outputs: 
% bR    = numerator 
% aR    = denominator 

% States: 
theta1  = theta(1); % (1) theta:  pitch angle response
% theta2  = theta(2); % (2) thetaD: pitch angle velocity


% Find the index for the discretized theta 
theta1N = wrapToPi(theta1); 

if abs(rad2deg(theta1N)) >= 95
    theta1N = pi - abs(theta1N); 
end 

thetaN = find(deg2rad(hydroCoeff.fineTheta) > abs(theta1N),1); 
% % Get transfer function coefficients depending on the discretized angle. 
aR       = zeros(1,7); 
bR       = zeros(1,7);

aR(1,:)    = aRInterp(:,thetaN);
bR(1,:)    = bRInterp(:,thetaN);


% % Get transfer function coefficients depending on the discretized angle. 
A       = zeros(6,6); 
B       = zeros(6,1); 
C       = zeros(1,6); 
D       = 0; 

[A(:,:), B(:,1), C(1,:), D(1)] = tf2ss(bR,aR);
